simulink model "Q2S"  (R2022a)
settings: Solver=VariableStepAuto  StartTime=0.0  StopTime=10.0  RelTol=1e-3
undefined symbols (not defined in the file or in its folder): sigbuilder_block
settings Model: Creator=Guilherme  LastModifiedBy=Guilherme

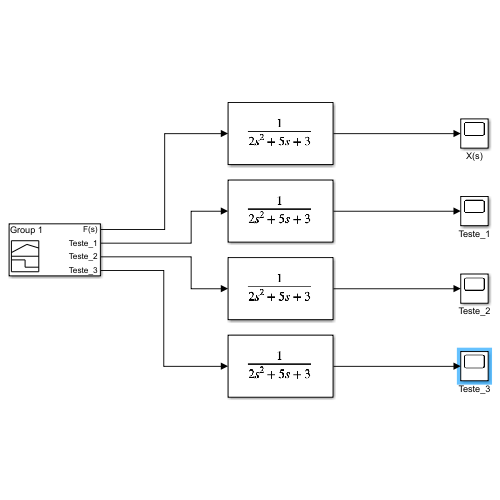
[thumbnail: Simulink's stored preview of the top-level diagram]
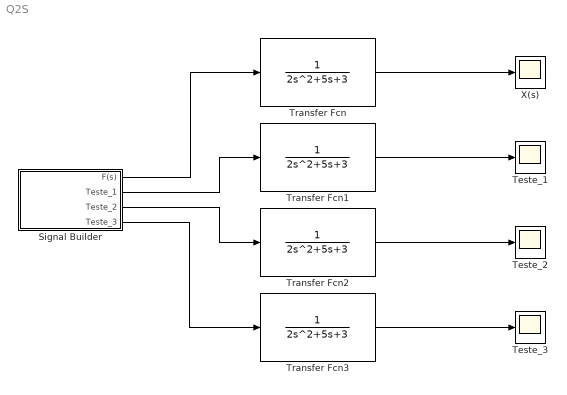
== system Q2S ==
  Signal Builder : Subsystem  Tag=STV Subsys  LoadFcn=sigbuilder_block('load');  StartFcn=sigbuilder_block('start');  StopFcn=sigbuilder_block('stop');  ClipboardFcn=sigbuilder_block('clipboard');  mask(Sigbuilder block){tuvar=[0:10]}
      mask help: Simulink:masks:SigbuilderBlock_MD
      mask init:
      | if ~strcmp(get_param(bdroot(gcbh),'SimulationStatus'),'stopped') tuvar = sigbuilder_block('maskInit'); end
      settings: CopyFcn=sigbuilder_block('copy');  DeleteFcn=sigbuilder_block('delete');  ModelCloseFcn=sigbuilder_block('modelClose');  PreSaveFcn=sigbuilder_block('preSave');  PauseFcn=sigbuilder_block('pause');  ContinueFcn=sigbuilder_block('continue');  NameChangeFcn=sigbuilder_block('namechange');  OpenFcn=sigbuilder_block('open',[141 173.4 550.8 400.2 ]);  CloseFcn=sigbuilder_block('close');
      mask Display: plot(0, 0, 100, 100,[2, 2, 32, 32, 2], [68, 8, 8, 68, 68],[32, 2], [38, 38], [32, 19, 2],[53, 60, 44], [32, 17, 17, 2],[16, 16, 31, 31]);txt = getActiveGroup(gcbh);text(2, 100, txt,'verticalAlignment', 'top');
  Teste_1 : Scope
  Teste_2 : Scope
  Teste_3 : Scope
  Transfer Fcn{,1..3} (4 alike) : TransferFcn  Denominator=[2 5 3]
  X(s) : Scope
  wires:
  Signal Builder/1(F(s)) -> Transfer Fcn/1
  Signal Builder/2(Teste_1) -> Transfer Fcn1/1
  Signal Builder/3(Teste_2) -> Transfer Fcn2/1
  Signal Builder/4(Teste_3) -> Transfer Fcn3/1
  Transfer Fcn/1 -> X(s)/1
  Transfer Fcn1/1 -> Teste_1/1
  Transfer Fcn2/1 -> Teste_2/1
  Transfer Fcn3/1 -> Teste_3/1

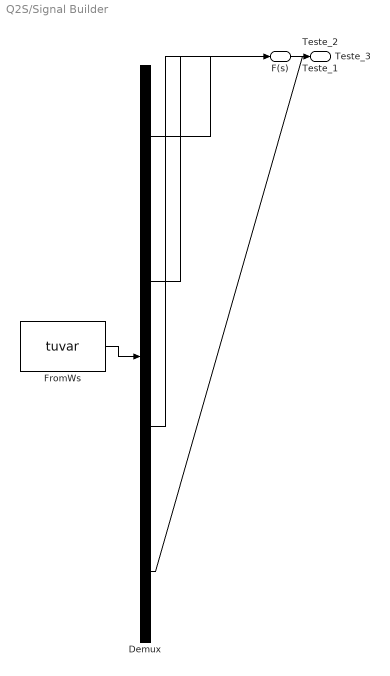
== system Q2S/Signal Builder ==
  Demux : Demux  Tag=STV Demux
      settings: DisplayOption=none
  FromWs : FromWorkspace  Tag=STV FromWs  VariableName=tuvar
      SigBuilderData=|
      | common.afterFinalStr = 'Extrapolate'
      | common.sampleTime = 0
      | dataSet.timeRange = [0 10]
      | dataSet.name = 'Group 1'
      | sbobj.Groups.Name = 'Group 1'
      | sbobj.Groups.Signals(1).Name = 'F(s)'
      | sbobj.Groups.Signals(1).XData = [0 5 5 10]
      | sbobj.Groups.Signals(1).YData = [2 2 0 0]
      | sbobj.Groups.Signals(2).Name = 'Teste_1'
      | sbobj.Groups.Signals(2).XData = [0 1 1 10]
      | sbobj.Groups.Signals(2).YData = [1 1 0 0]
      | sbobj.Groups.Signals(3).Name = 'Teste_2'
      | sbobj.Groups.Signals(3).XData = [0 0.1 0.1 10]
      | sbobj.Groups.Signals(3).YData = [10 10 0 0]
      | sbobj.Groups.Signals(4).Name = 'Teste_3'
      | sbobj.Groups.Signals(4).XData = [0 0.01 0.01 10]
      | sbobj.Groups.Signals(4).YData = [100 100 0 0]
  F(s) : Outport  Tag=STV Outport
  Teste_1 : Outport  Tag=STV Outport  Port=2
  Teste_2 : Outport  Tag=STV Outport  Port=3
  Teste_3 : Outport  Tag=STV Outport  Port=4
  wires:
  Demux/1 -> F(s)/1
  FromWs/1 -> Demux/1
  Demux/2 -> Teste_1/1
  Demux/3 -> Teste_2/1
  Demux/4 -> Teste_3/1
